simulink model "Problem3"  (R2020a)
settings: Solver=ode45  StartTime=0.0  StopTime=25.0  RelTol=1e-3
undefined symbols (not defined in the file): ctrl, g, I, Kf, m, mu, PBmax, Rr, slip, v0
settings Model: Creator=HP  LastModifiedBy=HP

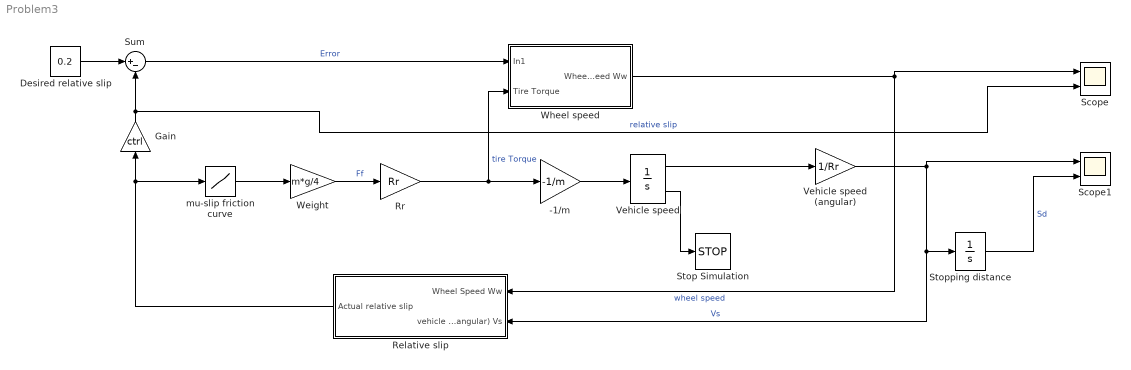
== system Problem3 ==
  -1/m : Gain  Gain=-1/m  SaturateOnIntegerOverflow=on  OutDataTypeStr=Inherit: Same as input  ParamDataTypeStr=Inherit: Same as input
  Desired relative slip : Constant  Value=0.2
  Gain : Gain  Gain=ctrl
  Relative slip : Subsystem
  Rr : Gain  Gain=Rr  SaturateOnIntegerOverflow=on  OutDataTypeStr=Inherit: Same as input  ParamDataTypeStr=Inherit: Same as input
  Scope : Scope  NumInputPorts=2
  Scope1 : Scope  NumInputPorts=2
  Stop Simulation : Stop
  Stopping distance : Integrator  UpperSaturationLimit=1000  LowerSaturationLimit=0
  Sum : Sum  Inputs=|+-
  Vehicle speed : Integrator  InitialCondition=v0  LimitOutput=on  UpperSaturationLimit=1000  LowerSaturationLimit=0  ShowSaturationPort=on
  Vehicle speed (angular) : Gain  Gain=1/Rr  SaturateOnIntegerOverflow=on  OutDataTypeStr=Inherit: Same as input  ParamDataTypeStr=Inherit: Same as input
  Weight : Gain  Gain=m*g/4  SaturateOnIntegerOverflow=on  OutDataTypeStr=Inherit: Same as input  ParamDataTypeStr=Inherit: Same as input
  Wheel speed : Subsystem
  mu-slip friction curve : Lookup_n-D  NumberOfTableDimensions=1  BreakpointsForDimension1=slip  Table=mu  SaturateOnIntegerOverflow=on  InputSameDT=on
  wires:
  Sum/1 -> Wheel speed/1(In1)  "Error"
  Rr/1 -> Wheel speed/2(Tire Torque), -1/m/1  "tire Torque"
  Wheel speed/1(Wheel Speed Ww) -> Scope/1, Relative slip/1(Wheel Speed Ww)  "wheel speed"
  Desired relative slip/1 -> Sum/1
  Gain/1 -> Scope/2, Sum/2  "relative slip"
  Relative slip/1(Actual relative slip) -> mu-slip friction curve/1, Gain/1
  mu-slip friction curve/1 -> Weight/1
  Weight/1 -> Rr/1  "Ff"
  -1/m/1 -> Vehicle speed/1
  Vehicle speed/2 -> Stop Simulation/1
  Vehicle speed/1 -> Vehicle speed (angular)/1
  Vehicle speed (angular)/1 -> Scope1/1, Stopping distance/1, Relative slip/2(vehicle speed (angular) Vs)  "Vs"
  Stopping distance/1 -> Scope1/2  "Sd"

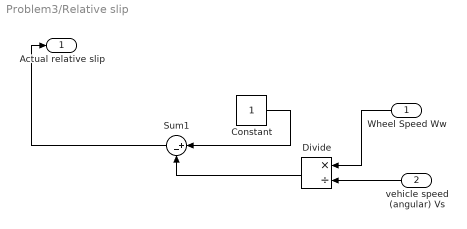
== system Problem3/Relative slip ==
  Wheel Speed Ww : Inport
  vehicle speed (angular) Vs : Inport  Port=2
  Constant : Constant
  Divide : Product  Inputs=*/
  Sum1 : Sum  Inputs=|+-
  Actual relative slip : Outport
  wires:
  Sum1/1 -> Actual relative slip/1
  Constant/1 -> Sum1/1
  vehicle speed (angular) Vs/1 -> Divide/2
  Divide/1 -> Sum1/2
  Wheel Speed Ww/1 -> Divide/1

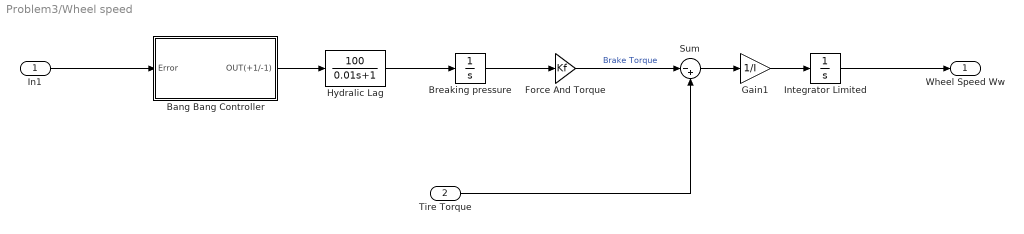
== system Problem3/Wheel speed ==
  In1 : Inport
  Tire Torque : Inport  Port=2
  Bang Bang Controller : Subsystem
  Breaking pressure : Integrator  LimitOutput=on  UpperSaturationLimit=PBmax  LowerSaturationLimit=0
  Force And Torque : Gain  Gain=Kf
  Gain1 : Gain  Gain=1/I
  Hydralic Lag : TransferFcn  Numerator=[100]  Denominator=[0.01 1]
  Integrator Limited : Integrator  InitialCondition=v0/Rr  LimitOutput=on  UpperSaturationLimit=1000  LowerSaturationLimit=0
  Sum : Sum  Inputs=|-+
  Wheel Speed Ww : Outport
  wires:
  In1/1 -> Bang Bang Controller/1(Error)
  Breaking pressure/1 -> Force And Torque/1
  Tire Torque/1 -> Sum/2
  Sum/1 -> Gain1/1
  Integrator Limited/1 -> Wheel Speed Ww/1
  Gain1/1 -> Integrator Limited/1
  Hydralic Lag/1 -> Breaking pressure/1
  Force And Torque/1 -> Sum/1  "Brake Torque"
  Bang Bang Controller/1(OUT(+1/-1)) -> Hydralic Lag/1

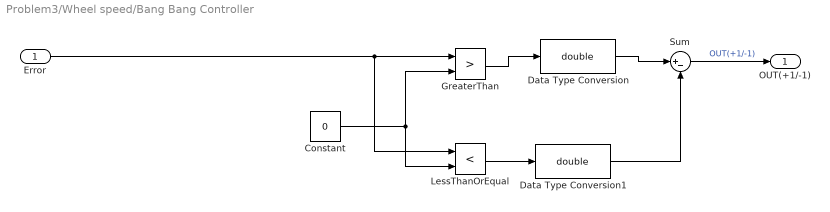
== system Problem3/Wheel speed/Bang Bang Controller ==
  Error : Inport
  Constant : Constant  Value=0
  Data Type Conversion : DataTypeConversion  OutDataTypeStr=double  RndMeth=Zero
  Data Type Conversion1 : DataTypeConversion  OutDataTypeStr=double  RndMeth=Zero
  GreaterThan : RelationalOperator  Operator=>  OutDataTypeStr=boolean  RndMeth=Simplest
  LessThanOrEqual : RelationalOperator  Operator=<  OutDataTypeStr=boolean  RndMeth=Simplest
  Sum : Sum  Inputs=|+-
  OUT(+1/-1) : Outport
  wires:
  GreaterThan/1 -> Data Type Conversion/1
  Error/1 -> LessThanOrEqual/1, GreaterThan/1
  Constant/1 -> GreaterThan/2, LessThanOrEqual/2
  LessThanOrEqual/1 -> Data Type Conversion1/1
  Data Type Conversion/1 -> Sum/1
  Data Type Conversion1/1 -> Sum/2
  Sum/1 -> OUT(+1/-1)/1  "OUT(+1/-1)"
